simulink model "Planta_ReactorAgitado_Permanente_2017a"  (R2017a)
settings: Solver=VariableStepAuto  StartTime=0.0  StopTime=120  RelTol=1e-3  EnableMultiTasking=on
undefined symbols (not defined in the file or in its folder): Da1, Da2
settings Model: Creator=Jesús Lopez  LastModifiedBy=jesus
settings OptimizationCC: LifeSpan=inf
settings DebuggingCC: SFUnexpectedBacktrackingDiag=warning  SFNoUnconditionalDefaultTransitionDiag=warning  SFExecutionAtInitializationDiag=none
settings GRTTargetCC: TargetLangStandard=C89/C90 (ANSI)  GeneratePreprocessorConditionals=Disable all
settings ConfigComp: CovMetricSettings=dw  CovHtmlReporting=on  CovSaveCumulativeToWorkspaceVar=on  CovSaveSingleToWorkspaceVar=on  CovExternalEMLEnable=off

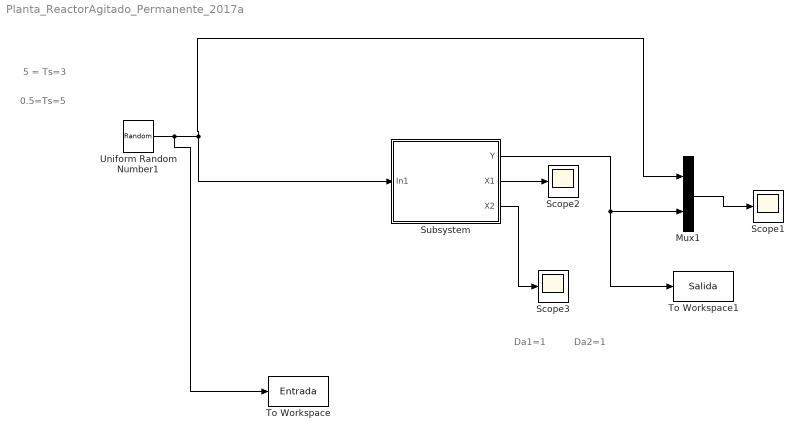
== system Planta_ReactorAgitado_Permanente_2017a ==
  note: 0.5=Ts=5
  note: 5 = Ts=3
  note: Da1=1
  note: Da2=1
  Mux1 : Mux  Inputs=2
  Scope1 : Scope
  Scope2 : Scope
  Scope3 : Scope
  Subsystem : Subsystem
  To Workspace : ToWorkspace  VariableName=Entrada  SampleTime=0.06
  To Workspace1 : ToWorkspace  VariableName=Salida  SampleTime=0.06
  Uniform Random Number1 : UniformRandomNumber  Minimum=0.5  Maximum=5  SampleTime=6
  wires:
  Uniform Random Number1/1 -> Subsystem/1(In1), Mux1/1, To Workspace/1
  Mux1/1 -> Scope1/1
  Subsystem/1(Y) -> To Workspace1/1, Mux1/2
  Subsystem/2(X1) -> Scope2/1
  Subsystem/3(X2) -> Scope3/1

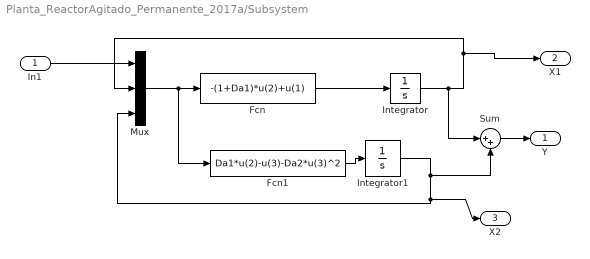
== system Planta_ReactorAgitado_Permanente_2017a/Subsystem ==
  In1 : Inport
  Fcn : Fcn  Expr=-(1+Da1)*u(2)+u(1)
  Fcn1 : Fcn  Expr=Da1*u(2)-u(3)-Da2*u(3)^2
  Integrator : Integrator
  Integrator1 : Integrator
  Mux : Mux  Inputs=3
  Sum : Sum  Inputs=|++
  Y : Outport
  X1 : Outport  Port=2
  X2 : Outport  Port=3
  wires:
  In1/1 -> Mux/1
  Fcn1/1 -> Integrator1/1
  Mux/1 -> Fcn1/1, Fcn/1
  Fcn/1 -> Integrator/1
  Integrator/1 -> Sum/1, X1/1, Mux/2
  Integrator1/1 -> Sum/2, X2/1, Mux/3
  Sum/1 -> Y/1
